simulink model "ballandplatesim"  (Simulink 5.1)
settings: Solver=ode45  StartTime=0.0  StopTime=stoptime  RelTol=1e-3
libraries: mpt_sim x4, simulink x1
settings Model: LastModifiedBy=michal  BooleanDataType=on

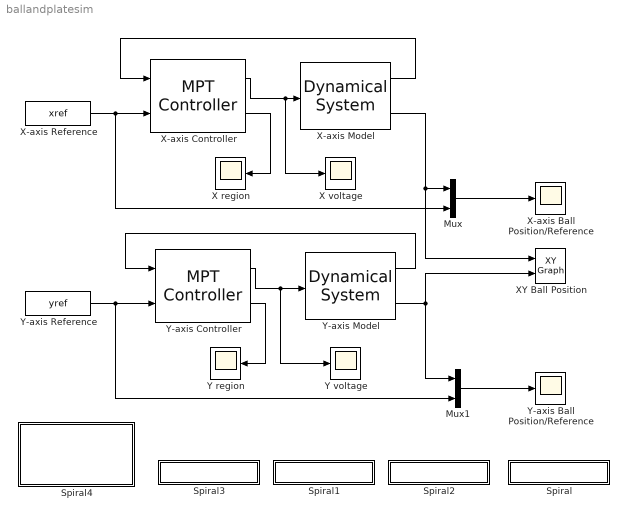
== system ballandplatesim ==
  Mux : Mux  Inputs=2
  Mux1 : Mux  Inputs=2
  Spiral : Subsystem  SimViewingDevice=off
      settings: OpenFcn=load kreisvolvente_1  Permissions=ReadWrite  RTWFcnNameOpts=Auto  RTWFileNameOpts=Auto
      mask Display: disp('Spiral')
  Spiral1 : Subsystem  SimViewingDevice=off
      settings: OpenFcn=load quadrat_20  Permissions=ReadWrite  RTWFcnNameOpts=Auto  RTWFileNameOpts=Auto
      mask Display: disp('Box')
  Spiral2 : Subsystem  SimViewingDevice=off
      settings: OpenFcn=load circle_10  Permissions=ReadWrite  RTWFcnNameOpts=Auto  RTWFileNameOpts=Auto
      mask Display: disp('Circle')
  Spiral3 : Subsystem  SimViewingDevice=off
      settings: OpenFcn=load star_40  Permissions=ReadWrite  RTWFcnNameOpts=Auto  RTWFileNameOpts=Auto
      mask Display: disp('Star')
  Spiral4 : Subsystem  SimViewingDevice=off
      settings: OpenFcn=ballandplate  Permissions=ReadWrite  RTWFcnNameOpts=Auto  RTWFileNameOpts=Auto
      mask Display: fprintf('Load parameters\nand controller')
  X region : Scope
      settings: TimeRange=25  YMin=0  YMax=300  SaveToWorkspace=off  SaveName=ScopeData4  LimitDataPoints=on  MaxDataPoints=5000
  X voltage : Scope
      settings: TimeRange=25  YMin=-20  YMax=20  SaveToWorkspace=off  SaveName=ScopeData2  LimitDataPoints=on  MaxDataPoints=5000
  X-axis Ball Position/Reference : Scope
      settings: TimeRange=25  YMin=-20  YMax=20  SaveToWorkspace=off  SaveName=ScopeData  LimitDataPoints=on  MaxDataPoints=5000
  X-axis Controller : mpt_sim/MPT Controller  ctrl=ecx  Ts=[]  infbreak=on
  X-axis Model : mpt_sim/Dynamical System  sysStruct=sysx  x0=[0;0;0;0]  Ts=[]  constr=on
  X-axis Reference : FromWorkspace  VariableName=xref  SampleTime=0.03  OutputAfterFinalValue=Extrapolation
  XY Ball Position : simulink/Sinks/XY Graph  xmin=-30  xmax=30  ymin=-30  ymax=30  st=-1
  Y region : Scope
      settings: TimeRange=25  YMin=0  YMax=300  SaveToWorkspace=off  SaveName=ScopeData5  LimitDataPoints=on  MaxDataPoints=5000
  Y voltage : Scope
      settings: TimeRange=25  YMin=-20  YMax=20  SaveToWorkspace=off  SaveName=ScopeData3  LimitDataPoints=on  MaxDataPoints=5000
  Y-axis Ball Position/Reference : Scope
      settings: TimeRange=25  YMin=-20  YMax=20  SaveToWorkspace=off  LimitDataPoints=on  MaxDataPoints=5000
  Y-axis Controller : mpt_sim/MPT Controller  ctrl=ecy  Ts=[]  infbreak=on
  Y-axis Model : mpt_sim/Dynamical System  sysStruct=sysy  x0=[0;0;0;0]  Ts=[]  constr=on
  Y-axis Reference : FromWorkspace  VariableName=yref  SampleTime=0.03  OutputAfterFinalValue=Extrapolation
  wires:
  X-axis Model/1 -> X-axis Controller/1
  X-axis Model/2 -> XY Ball Position/1, Mux/1
  Mux/1 -> X-axis Ball Position/Reference/1
  X-axis Controller/1 -> X-axis Model/1, X voltage/1
  X-axis Reference/1 -> X-axis Controller/2, Mux/2
  Y-axis Reference/1 -> Y-axis Controller/2, Mux1/2
  Y-axis Controller/1 -> Y-axis Model/1, Y voltage/1
  Y-axis Model/1 -> Y-axis Controller/1
  Y-axis Model/2 -> Mux1/1, XY Ball Position/2
  Mux1/1 -> Y-axis Ball Position/Reference/1
  X-axis Controller/2 -> X region/1
  Y-axis Controller/2 -> Y region/1

== system ballandplatesim/Spiral ==

== system ballandplatesim/Spiral1 ==

== system ballandplatesim/Spiral2 ==

== system ballandplatesim/Spiral3 ==

== system ballandplatesim/Spiral4 ==
